simulink model "haul_truck"  (R2024b)
settings: Solver=VariableStepAuto  StartTime=0.0  StopTime=1000  RelTol=1e-3
undefined symbols (not defined in the file or in its folder): DiscIntNeverNeededParam
libraries: SignalEditorBlockLib x3, slpidlib x1
settings Model: Creator=Ergin  LastModifiedBy=Ergin

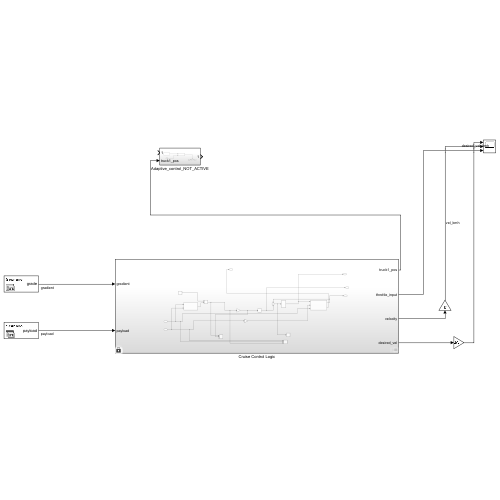
[thumbnail: Simulink's stored preview of the top-level diagram]
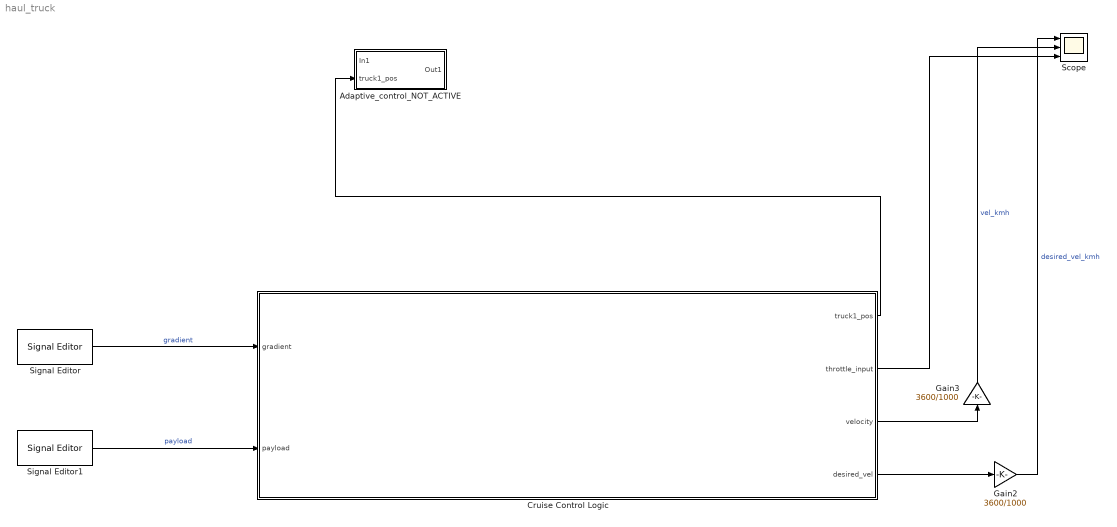
== system haul_truck ==
  Adaptive_control_NOT_ACTIVE : Subsystem
  Cruise Control Logic : Subsystem
  Gain2 : Gain  Gain=3600/1000
  Gain3 : Gain  Gain=3600/1000
  Scope : Scope  NumInputPorts=3
  Signal Editor : SignalEditorBlockLib/Signal Editor  FileName=grade_signals.mat  ActiveScenario=Scenario  ActiveSignal=grade  IsBus=off  OutputBusObjectStr=Bus: BusObject  SampleTime=0  Interpolate=off  ZeroCross=off  OutputAfterFinalValue=Setting to zero  Unit=inherit  PreserveSignalName=on  ApplySigPropsToAllScenarios=on  ApplySigPropsToAllSignals=off
  Signal Editor1 : SignalEditorBlockLib/Signal Editor  FileName=payload_signals.mat  ActiveScenario=Scenario  ActiveSignal=payload  IsBus=off  OutputBusObjectStr=Bus: BusObject  SampleTime=0  Interpolate=off  ZeroCross=off  OutputAfterFinalValue=Setting to zero  Unit=inherit  PreserveSignalName=on  ApplySigPropsToAllScenarios=on  ApplySigPropsToAllSignals=off
  wires:
  Gain2/1 -> Scope/1  "desired_vel_kmh"
  Gain3/1 -> Scope/2  "vel_kmh"
  Signal Editor/1 -> Cruise Control Logic/1(gradient)  "gradient"
  Signal Editor1/1 -> Cruise Control Logic/2(payload)  "payload"
  Cruise Control Logic/2(throttle_input) -> Scope/3
  Cruise Control Logic/3(velocity) -> Gain3/1
  Cruise Control Logic/4(desired_vel) -> Gain2/1
  Cruise Control Logic/1(truck1_pos) -> Adaptive_control_NOT_ACTIVE/2(truck1_pos)

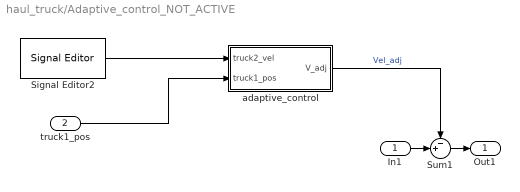
== system haul_truck/Adaptive_control_NOT_ACTIVE ==
  In1 : Inport
  truck1_pos : Inport  Port=2
  Signal Editor2 : SignalEditorBlockLib/Signal Editor  FileName=truck2_vel_signals.mat  ActiveScenario=Scenario  ActiveSignal=truck2_vel  IsBus=off  OutputBusObjectStr=Bus: BusObject  SampleTime=0  Interpolate=off  ZeroCross=off  OutputAfterFinalValue=Setting to zero  Unit=inherit  PreserveSignalName=on  ApplySigPropsToAllScenarios=on  ApplySigPropsToAllSignals=off
  Sum1 : Sum  Inputs=-+|
  adaptive_control : Subsystem
  Out1 : Outport
  wires:
  Signal Editor2/1 -> adaptive_control/1(truck2_vel)
  In1/1 -> Sum1/2
  adaptive_control/1(V_adj) -> Sum1/1  "Vel_adj"
  Sum1/1 -> Out1/1
  truck1_pos/1 -> adaptive_control/2(truck1_pos)

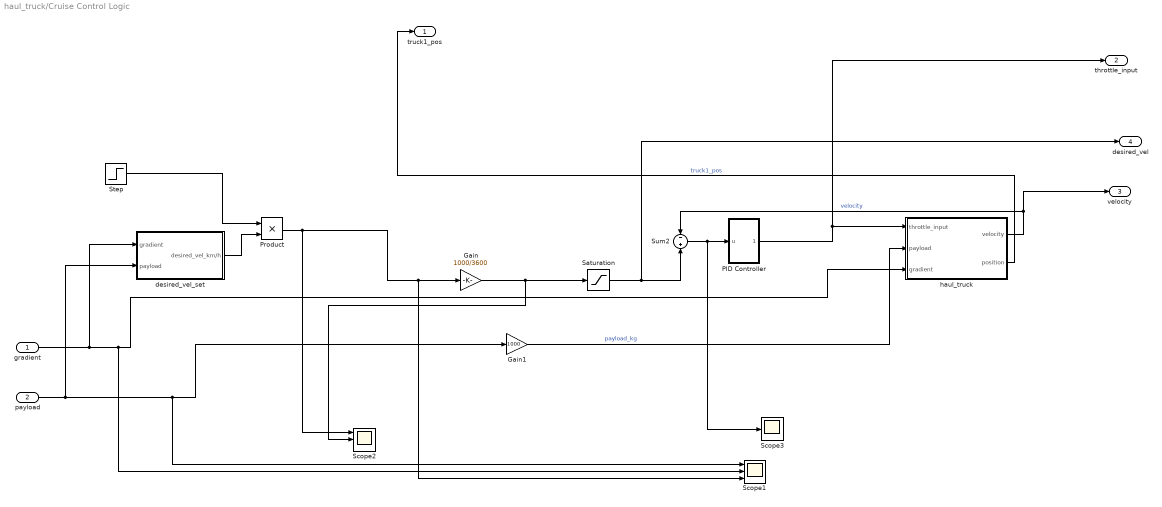
== system haul_truck/Cruise Control Logic ==
  gradient : Inport
  payload : Inport  Port=2
  Gain : Gain  Gain=1000/3600
  Gain1 : Gain  Gain=1000
  PID Controller : Subsystem
  Product : Product
  Saturation : Saturate  UpperLimit=1000000  LowerLimit=0
  Scope1 : Scope  NumInputPorts=3
  Scope2 : Scope  NumInputPorts=3
  Scope3 : Scope
  Step : Step  Time=10  SampleTime=0
  Sum2 : Sum  Inputs=-+
  desired_vel_set : Subsystem
  haul_truck : Subsystem
  truck1_pos : Outport
  throttle_input : Outport  Port=2
  velocity : Outport  Port=3
  desired_vel : Outport  Port=4
  wires:
  haul_truck/2(position) -> truck1_pos/1  "truck1_pos"
  haul_truck/1(velocity) -> velocity/1, Sum2/1  "velocity"
  gradient/1 -> Scope1/2, haul_truck/3(gradient), desired_vel_set/1(gradient)
  Product/1 -> Scope2/1, Scope1/3, Gain/1
  Gain1/1 -> haul_truck/2(payload)  "payload_kg"
  Saturation/1 -> desired_vel/1, Sum2/2
  Sum2/1 -> PID Controller/1(u), Scope3/1
  payload/1 -> Gain1/1, Scope1/1, desired_vel_set/2(payload)
  desired_vel_set/1(desired_vel_km/h) -> Product/2
  Gain/1 -> Saturation/1, Scope2/2
  Step/1 -> Product/1
  PID Controller/1(throttle_input) -> throttle_input/1, haul_truck/1(throttle_input)

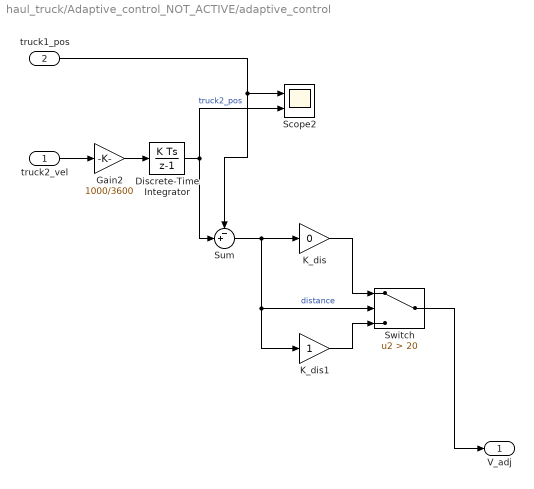
== system haul_truck/Adaptive_control_NOT_ACTIVE/adaptive_control ==
  truck2_vel : Inport
  truck1_pos : Inport  Port=2
  Discrete-Time Integrator : DiscreteIntegrator  InitialCondition=1  SampleTime=0.01  ICPrevOutput=DiscIntNeverNeededParam  ICPrevScaledInput=DiscIntNeverNeededParam
  Gain2 : Gain  Gain=1000/3600
  K_dis : Gain  Gain=0
  K_dis1 : Gain
  Scope2 : Scope  NumInputPorts=2
  Sum : Sum  Inputs=-+|
  Switch : Switch  Criteria=u2 > Threshold  Threshold=20  SaturateOnIntegerOverflow=off  InputSameDT=off
  V_adj : Outport
  wires:
  truck1_pos/1 -> Sum/1, Scope2/1
  Sum/1 -> K_dis1/1, Switch/2, K_dis/1  "distance"
  Discrete-Time Integrator/1 -> Sum/2, Scope2/2  "truck2_pos"
  K_dis/1 -> Switch/1
  Gain2/1 -> Discrete-Time Integrator/1
  K_dis1/1 -> Switch/3
  truck2_vel/1 -> Gain2/1
  Switch/1 -> V_adj/1

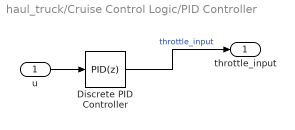
== system haul_truck/Cruise Control Logic/PID Controller ==
  u : Inport
  Discrete PID Controller : slpidlib/PID Controller  Controller=PID  Form=Parallel  TimeDomain=Discrete-time  UseExternalTs=off  SampleTime=-1  IntegratorMethod=Forward Euler  FilterMethod=Forward Euler  ControllerParametersSource=internal  P=10.2  I=8.321  UseKiTs=off  D=-0.2006  UseExternalDerivativeSource=off  N=4.365  UseFilter=on  TunerSelectOption=Transfer Function Based (PID Tuner App)  InitialConditionSource=internal  InitialConditionForIntegrator=0  InitialConditionForFilter=0  DifferentiatorICPrevScaledInput=0  ExternalReset=none  TrackingMode=off  Kt=1  LimitOutput=on  SatLimitsSource=internal  UpperSaturationLimit=100  LowerSaturationLimit=0  LinearizeAsGain=on  AntiWindupMode=clamping  Kb=1  LimitIntegrator=off  UpperIntegratorSaturationLimit=inf  LowerIntegratorSaturationLimit=-inf  POutMin=[]  POutMax=[]  IOutMin=[]  IOutMax=[]  DOutMin=[]  DOutMax=[]  NOutMin=[]  NOutMax=[]  SumOutMin=0  SumOutMax=100  SaturationOutMin=[]  SaturationOutMax=[]  PParamMin=[]  PParamMax=[]  IParamMin=[]  IParamMax=[]  DParamMin=[]  DParamMax=[]  NParamMin=[]  NParamMax=[]  KbParamMin=[]  KbParamMax=[]  KtParamMin=[]  KtParamMax=[]  KbOutMin=[]  KbOutMax=[]  KtOutMin=[]  KtOutMax=[]  IntegratorOutMin=[]  IntegratorOutMax=[]  FilterOutMin=[]  FilterOutMax=[]  SumI1OutMin=[]  SumI1OutMax=[]  SumI2OutMin=[]  SumI2OutMax=[]  SumI3OutMin=[]  SumI3OutMax=[]  SumI4OutMin=[]  SumI4OutMax=[]  SumDOutMin=[]  SumDOutMax=[]  DifferentiatorOutMin=[]  DifferentiatorOutMax=[]  FilterDiffOutCoefMin=[]  FilterDiffOutCoefMax=[]  ReciprocalOutMin=[]  ReciprocalOutMax=[]  SumDenOutMin=[]  SumDenOutMax=[]  SumNumOutMin=[]  SumNumOutMax=[]  DivideOutMin=[]  DivideOutMax=[]  UdiffTsProdOutMin=[]  UdiffTsProdOutMax=[]  NTsProdOutMin=[]  NTsProdOutMax=[]  UintegralTsProdOutMin=[]  UintegralTsProdOutMax=[]  UngainTsProdOutMin=[]  UngainTsProdOutMax=[]  ClampingZeroOutDataTypeStr=Inherit: Inherit via back propagation  ClampingZeroOutMin=[]  ClampingZeroOutMax=[]  FilterDenConstantOutDataTypeStr=Inherit: Inherit via back propagation  FilterDenConstantOutMin=[]  FilterDenConstantOutMax=[]  PCopyOutDataTypeStr=Inherit: Inherit via back propagation  PCopyOutMin=[]  PCopyOutMax=[]  NCopyOutDataTypeStr=Inherit: Inherit via back propagation  NCopyOutMin=[]  NCopyOutMax=[]  IntegratorContinuousStateAttributes=''  IntegratorStateMustResolveToSignalObject=off  IntegratorRTWStateStorageClass=Auto  FilterContinuousStateAttributes=''  FilterStateMustResolveToSignalObject=off  FilterRTWStateStorageClass=Auto  ParallelPVariant=InternalParameters  IdealPVariant=Disabled  IVariant=InternalParameters  DVariant=InternalParameters  IntegratorVariant=Discrete  SatVariant=Enabled  AWVariant=DiscClampingParallel  PCopyVariant=Disabled  TRVariant=Disabled  FdbkBlocksVariant=Forward  IdealPFdbkVariant=Disabled  SatFdbkVariant=Disabled  DerivativeFilterVariant=ForwardEulerFilter  NVariant=InternalParameters  NCopyVariant=Disabled  FilterICVariant=InternalICsFilter  IntegratorICVariant=InternalICs  ExternalResetVariant=Disabled  TRSumVariant=Passthrough  SumFdbkVariant=Disabled  SumVariant=Sum_PID  TsampFilterVariant=InternalTs  TsampNgainVariant=Passthrough  TsampIntegralVariant=Disabled_SignalSpec  ExternalSaturationOutDataTypeStr=Inherit: Same as second input  DerivativeSourceVariant=ErrorSignal  PreIntVariant=InternalPreInt
  throttle_input : Outport
  wires:
  u/1 -> Discrete PID Controller/1
  Discrete PID Controller/1 -> throttle_input/1  "throttle_input"

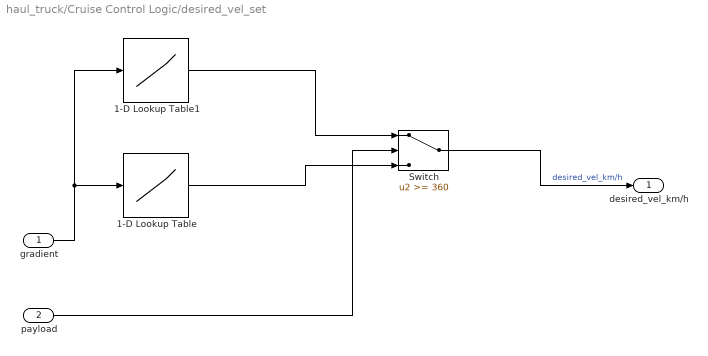
== system haul_truck/Cruise Control Logic/desired_vel_set ==
  gradient : Inport
  payload : Inport  Port=2
  1-D Lookup Table : Lookup_n-D  NumberOfTableDimensions=1  BreakpointsForDimension1=[-3;-2;-1;0;1;2;3]  Table=[30;40;50;60;55;50;45]  InternalRulePriority=Speed  RndMeth=Simplest
  1-D Lookup Table1 : Lookup_n-D  NumberOfTableDimensions=1  BreakpointsForDimension1=[-3;-2;-1;0;1;2;3]  Table=[20;25;30;45;40;35;25]  InternalRulePriority=Speed  RndMeth=Simplest
  Switch : Switch  Threshold=360  SaturateOnIntegerOverflow=off  InputSameDT=off
  desired_vel_km/h : Outport
  wires:
  gradient/1 -> 1-D Lookup Table/1, 1-D Lookup Table1/1
  Switch/1 -> desired_vel_km/h/1  "desired_vel_km/h"
  1-D Lookup Table/1 -> Switch/3
  1-D Lookup Table1/1 -> Switch/1
  payload/1 -> Switch/2

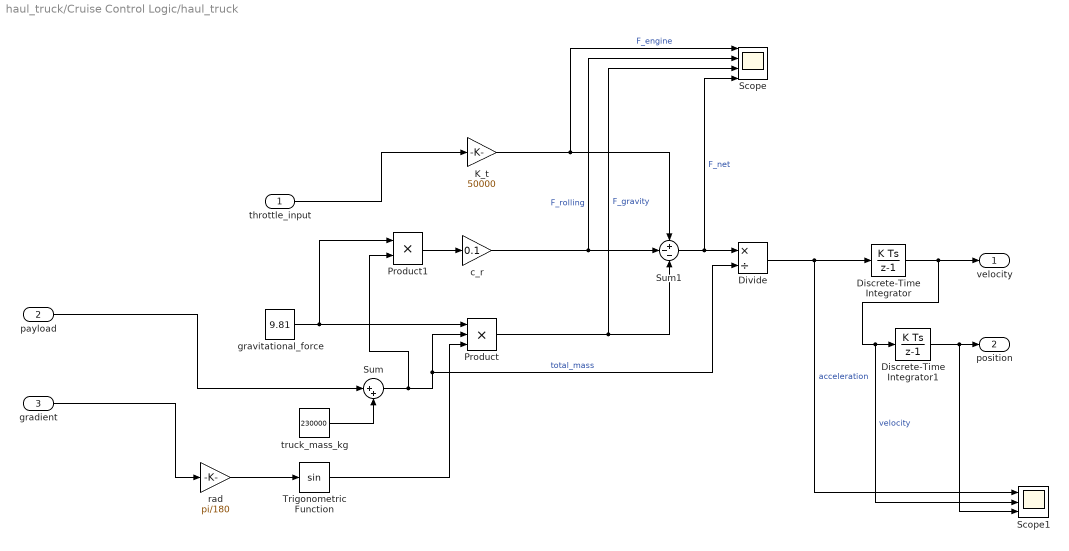
== system haul_truck/Cruise Control Logic/haul_truck ==
  throttle_input : Inport
  payload : Inport  Port=2
  gradient : Inport  Port=3
  Discrete-Time Integrator : DiscreteIntegrator  InitialCondition=1  SampleTime=0.01  ICPrevOutput=DiscIntNeverNeededParam  ICPrevScaledInput=DiscIntNeverNeededParam
  Discrete-Time Integrator1 : DiscreteIntegrator  InitialCondition=1  SampleTime=0.01  ICPrevOutput=DiscIntNeverNeededParam  ICPrevScaledInput=DiscIntNeverNeededParam
  Divide : Product  Inputs=*/
  K_t : Gain  Gain=50000
  Product : Product  Inputs=3
  Product1 : Product
  Scope : Scope  NumInputPorts=4
  Scope1 : Scope  NumInputPorts=3
  Sum : Sum  Inputs=|++
  Sum1 : Sum  Inputs=+--
  Trigonometric Function : Trigonometry
  c_r : Gain  Gain=0.1
  gravitational_force : Constant  Value=9.81  SampleTime=0.01
  rad : Gain  Gain=pi/180
  truck_mass_kg : Constant  Value=230000  SampleTime=0.01
  velocity : Outport
  position : Outport  Port=2
  wires:
  truck_mass_kg/1 -> Sum/2
  Trigonometric Function/1 -> Product/3
  Sum/1 -> Product1/2, Divide/2, Product/2  "total_mass"
  throttle_input/1 -> K_t/1
  K_t/1 -> Scope/1, Sum1/1  "F_engine"
  c_r/1 -> Scope/2, Sum1/2  "F_rolling"
  Sum1/1 -> Scope/4, Divide/1  "F_net"
  Divide/1 -> Scope1/1, Discrete-Time Integrator/1  "acceleration"
  Product/1 -> Scope/3, Sum1/3  "F_gravity"
  gravitational_force/1 -> Product1/1, Product/1
  Discrete-Time Integrator/1 -> Scope1/2, Discrete-Time Integrator1/1, velocity/1  "velocity"
  payload/1 -> Sum/1
  gradient/1 -> rad/1
  Discrete-Time Integrator1/1 -> Scope1/3, position/1
  Product1/1 -> c_r/1
  rad/1 -> Trigonometric Function/1
